simulink model "consumption_FrictionSimulation_v2"  (R2022a)
settings: Solver=FixedStepAuto  StartTime=0.0  StopTime=3.0  FixedStep=1e-6  RelTol=1e-3
values from neighbouring files (symbols this model uses):
  duckMass = 0.0708    [consumptionTorqueSimWS.mat]
  duckWeight = 0.0708    [consumptionTorqueSimWS.mat]
  forcePeriod = 0.2    [consumptionTorqueSimWS.mat]
  forcePulseWidthPercent = 99    [consumptionTorqueSimWS.mat]
  momentArmLength = 0.0635    [consumptionTorqueSimWS.mat]
  phase0 = 0    [consumptionTorqueSimWS.mat]
  phase1 = 0    [consumptionTorqueSimWS.mat]
  phase2 = 0    [consumptionTorqueSimWS.mat]
undefined symbols (not defined in the file or in its folder): coeffFriction
libraries: simulink x3
settings Model: Creator=natha  LastModifiedBy=fnalheji42
settings DebuggingCC: UnconnectedInputMsg=warning  UnconnectedOutputMsg=warning  UnconnectedLineMsg=warning
settings RTWCC: DLArmComputeVersion=19.05

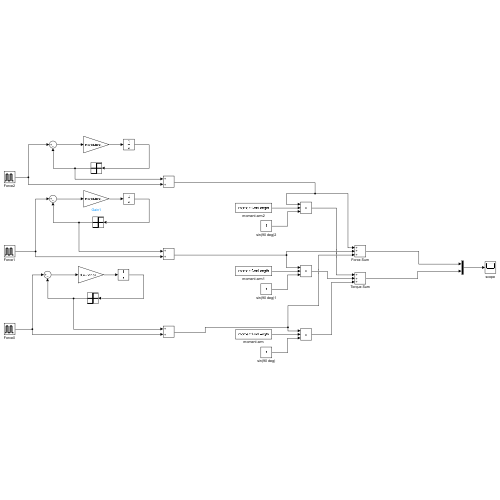
[thumbnail: Simulink's stored preview of the top-level diagram]
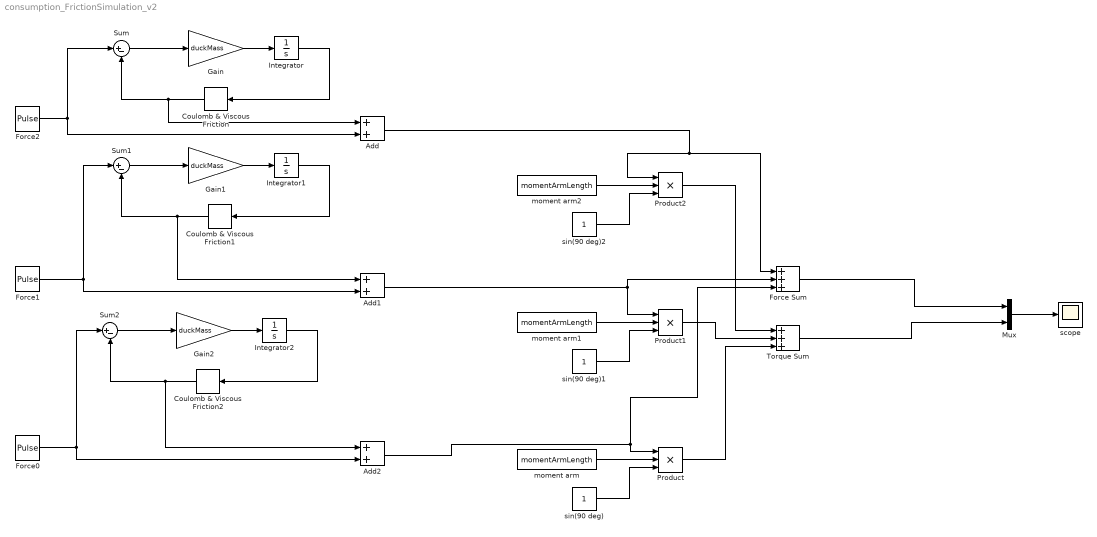
== system consumption_FrictionSimulation_v2 ==
  Add : Sum
  Add1 : Sum
  Add2 : Sum
  Coulomb & Viscous Friction : simulink/Discontinuities/Coulomb & Viscous Friction  offset=duckMass*9.8*coeffFriction  gain=0
  Coulomb & Viscous Friction1 : simulink/Discontinuities/Coulomb & Viscous Friction  offset=duckMass*9.8*coeffFriction  gain=0
  Coulomb & Viscous Friction2 : simulink/Discontinuities/Coulomb & Viscous Friction  offset=duckMass*9.8*coeffFriction  gain=0
  Force Sum : Sum  Inputs=+++
  Force0 : DiscretePulseGenerator  PulseType=Time based  Amplitude=9.8*duckWeight  Period=forcePeriod  PulseWidth=forcePulseWidthPercent  PhaseDelay=phase0
  Force1 : DiscretePulseGenerator  PulseType=Time based  Amplitude=9.8*duckWeight  Period=forcePeriod  PulseWidth=forcePulseWidthPercent  PhaseDelay=phase1
  Force2 : DiscretePulseGenerator  PulseType=Time based  Amplitude=9.8*duckWeight  Period=forcePeriod  PulseWidth=forcePulseWidthPercent  PhaseDelay=phase2
  Gain : Gain  Gain=duckMass
  Gain1 : Gain  Gain=duckMass
  Gain2 : Gain  Gain=duckMass
  Integrator : Integrator
  Integrator1 : Integrator
  Integrator2 : Integrator
  Mux : Mux  Inputs=2
  Product : Product  Inputs=3
  Product1 : Product  Inputs=3
  Product2 : Product  Inputs=3
  Sum : Sum  Inputs=|+-
  Sum1 : Sum  Inputs=|+-
  Sum2 : Sum  Inputs=|+-
  Torque Sum : Sum  Inputs=+++
  moment arm : Constant  Value=momentArmLength
  moment arm1 : Constant  Value=momentArmLength
  moment arm2 : Constant  Value=momentArmLength
  scope : Scope
  sin(90 deg) : Constant
  sin(90 deg)1 : Constant
  sin(90 deg)2 : Constant
  wires:
  Product/1 -> Torque Sum/3
  sin(90 deg)/1 -> Product/3
  moment arm/1 -> Product/2
  Product1/1 -> Torque Sum/2
  sin(90 deg)1/1 -> Product1/3
  moment arm1/1 -> Product1/2
  Product2/1 -> Torque Sum/1
  sin(90 deg)2/1 -> Product2/3
  moment arm2/1 -> Product2/2
  Add/1 -> Product2/1, Force Sum/1
  Mux/1 -> scope/1
  Torque Sum/1 -> Mux/2
  Force Sum/1 -> Mux/1
  Sum/1 -> Gain/1
  Gain/1 -> Integrator/1
  Integrator/1 -> Coulomb & Viscous Friction/1
  Coulomb & Viscous Friction/1 -> Add/1, Sum/2
  Integrator1/1 -> Coulomb & Viscous Friction1/1
  Sum1/1 -> Gain1/1
  Gain1/1 -> Integrator1/1
  Coulomb & Viscous Friction1/1 -> Sum1/2, Add1/1
  Force2/1 -> Add/2, Sum/1
  Force1/1 -> Add1/2, Sum1/1
  Add1/1 -> Force Sum/2, Product1/1
  Add2/1 -> Force Sum/3, Product/1
  Coulomb & Viscous Friction2/1 -> Add2/1, Sum2/2
  Integrator2/1 -> Coulomb & Viscous Friction2/1
  Gain2/1 -> Integrator2/1
  Sum2/1 -> Gain2/1
  Force0/1 -> Sum2/1, Add2/2
